simulink model "PV_MPPT"  (Simulink 10.0)
settings: Solver=ode23s  StartTime=0.0  StopTime=10  RelTol=1e-3  EnableMultiTasking=on
libraries: powerlib x12, powerlib_extras x2, simulink x1
settings Model: Creator=Administrator  LastModifiedBy=bhisma
settings SolverCC: ZeroCrossAlgorithm=Non-adaptive
settings DataIOCC: LimitDataPoints=on  SignalLoggingSaveFormat=ModelDataLogs
settings OptimizationCC: ExpressionDepthLimit=2147483647  InitFltsAndDblsToZero=on
settings DebuggingCC: SaveWithParameterizedLinksMsg=none  SolverPrmCheckMsg=warning  FcnCallInpInsideContextMsg=warning  StateNameClashWarn=warning
settings SFSimCC: SimUseLocalCustomCode=on  SimParseCustomCode=off  CustomCodeUndefinedFunction=FilterOut
settings RTWCC: RTWUseLocalCustomCode=on

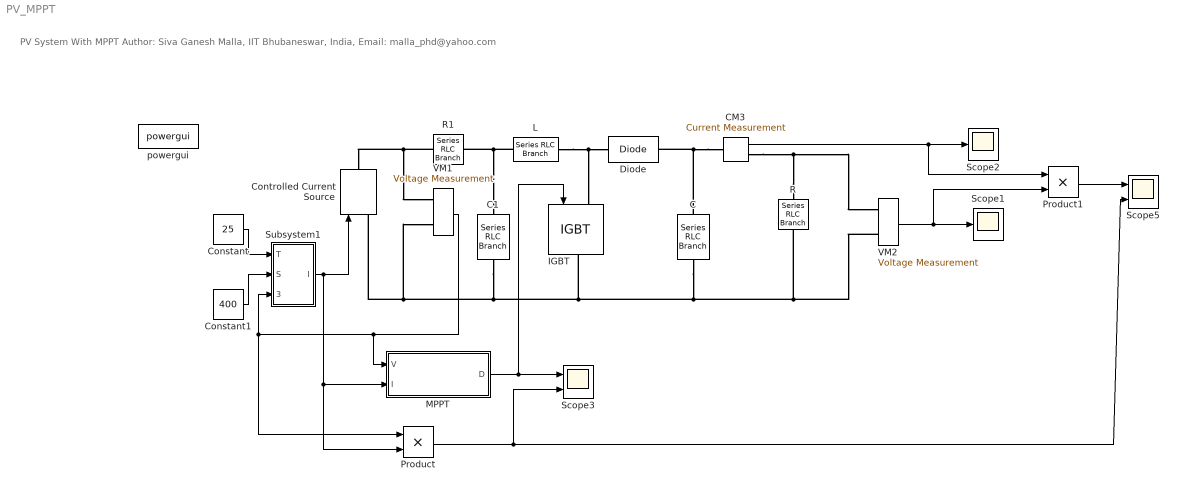
== system PV_MPPT ==
  note: PV System With MPPT
      | Author: Siva Ganesh Malla, IIT Bhubaneswar, India, Email: malla_phd@yahoo.com
  C : powerlib/Elements/Series RLC Branch  PhysicalDomain=powersysdomain  SubClassName=unknown  LeftPortType=p1  RightPortType=p1  LConnTagsString=__new0  RConnTagsString=__new0  BranchType=C  Resistance=0.01  Inductance=1.0  SetiL0=off  InitialCurrent=0  Capacitance=2e-3  Setx0=off  InitialVoltage=200  Measurements=None
      settings: SourceProductName=Simscape Electrical
  C1 : powerlib/Elements/Series RLC Branch  PhysicalDomain=powersysdomain  SubClassName=unknown  LeftPortType=p1  RightPortType=p1  LConnTagsString=__new0  RConnTagsString=__new0  BranchType=C  Resistance=0.01  Inductance=1.0  SetiL0=off  InitialCurrent=0  Capacitance=2e-3  Setx0=off  InitialVoltage=0  Measurements=None
      settings: SourceProductName=Simscape Electrical
  CM3 : powerlib/Measurements/Current Measurement  Tag=PoWeRsYsTeMmEaSuReMeNt  SystemSampleTime=-1  PhasorSimulation=off  OutputType=Magnitude  PSBequivalent=0
      settings: SourceProductName=Simscape Electrical
  Constant : Constant  Value=25
  Constant1 : Constant  Value=400
  Controlled Current Source : powerlib/Electrical Sources/Controlled Current Source  SystemSampleTime=-1  Initialize=on  Source_Type=AC  Amplitude=0  Phase=0  Frequency=0  Measurements=None
      settings: SourceProductName=Simscape Electrical
  Diode : powerlib/Power Electronics/Diode  SystemSampleTime=-1  Ron=0.001  Lon=0  Vf=0.8  IC=0  UseSnubber=off  Rs=500  Cs=250e-9  Measurements=off
      settings: SourceProductName=Simscape Electrical
  IGBT : powerlib/Power Electronics/IGBT  SystemSampleTime=-1  Ron=0.001  Lon=0  Vf=1  Tf=1e-6  Tt=2e-6  IC=0  Rs=1e5  Cs=inf  Measurements=off
      settings: SourceProductName=Simscape Electrical
  L : powerlib/Elements/Series RLC Branch  PhysicalDomain=powersysdomain  SubClassName=unknown  LeftPortType=p1  RightPortType=p1  LConnTagsString=__new0  RConnTagsString=__new0  BranchType=L  Resistance=1.0  Inductance=0.01  SetiL0=off  InitialCurrent=0  Capacitance=1.0  Setx0=off  InitialVoltage=0  Measurements=None
      settings: SourceProductName=Simscape Electrical
  MPPT : Subsystem
  Product : Product  RndMeth=Zero
  Product1 : Product  RndMeth=Zero
  R : powerlib/Elements/Series RLC Branch  PhysicalDomain=powersysdomain  SubClassName=unknown  LeftPortType=p1  RightPortType=p1  LConnTagsString=__new0  RConnTagsString=__new0  BranchType=R  Resistance=500  Inductance=1.0  SetiL0=off  InitialCurrent=0  Capacitance=1.0  Setx0=off  InitialVoltage=0  Measurements=None
      settings: SourceProductName=Simscape Electrical
  R1 : powerlib/Elements/Series RLC Branch  PhysicalDomain=powersysdomain  SubClassName=unknown  LeftPortType=p1  RightPortType=p1  LConnTagsString=__new0  RConnTagsString=__new0  BranchType=R  Resistance=1  Inductance=1.0  SetiL0=off  InitialCurrent=0  Capacitance=1.0  Setx0=off  InitialVoltage=0  Measurements=None
      settings: SourceProductName=Simscape Electrical
  Scope1 : Scope
  Scope2 : Scope
  Scope3 : Scope  NumInputPorts=2
  Scope5 : Scope  NumInputPorts=2
  Subsystem1 : Subsystem
  VM1 : powerlib/Measurements/Voltage Measurement  Tag=PoWeRsYsTeMmEaSuReMeNt  SystemSampleTime=-1  PhasorSimulation=off  OutputType=Magnitude  PSBequivalent=0
      settings: SourceProductName=Simscape Electrical
  VM2 : powerlib/Measurements/Voltage Measurement  Tag=PoWeRsYsTeMmEaSuReMeNt  SystemSampleTime=-1  PhasorSimulation=off  OutputType=Magnitude  PSBequivalent=0
      settings: SourceProductName=Simscape Electrical
  powergui : powerlib/powergui  SystemSampleTime=-1  SimulationMode=Continuous  SampleTime=50e-6  frequency=60  SPID=off  SwTol=0  Interpol=off  x0status=blocks  echomessages=off  HookPort=off  FunctionMessages=off  EnableUseOfTLC=off  RestoreLinks=warning  frequencyindice=0  Frange=[0:2:500]  Ylog=off  Xlog=on  ShowGrid=off  save=off  variable=ZData  ZoomFFT=on  StartTime=0.0  cycles=1  DisplayStyle=1  fundamental=60  FreqAxis=off  MaxFrequency=1000  frequencyindicesteady=1  RmsSteady=1  display=off  Ts=0  methode=off
      settings: SourceProductName=Simscape Electrical
  wires:
  Constant/1 -> Subsystem1/1(T)
  Subsystem1/1(I) -> Controlled Current Source/1, MPPT/2(I), Product/2
  CM3/1 -> Scope2/1, Product1/1
  VM2/1 -> Scope1/1, Product1/2
  VM1/1 -> Subsystem1/3(Uout), Product/1, MPPT/1(V)
  Product/1 -> Scope3/2, Scope5/2
  MPPT/1(D) -> IGBT/1, Scope3/1
  Constant1/1 -> Subsystem1/2(S)
  Product1/1 -> Scope5/1
  connections:
  C/RConn1 -- VM2/LConn2 -- R/RConn1 -- IGBT/RConn1 -- C1/RConn1 -- Controlled Current Source/LConn1 -- VM1/LConn2
  CM3/LConn1 -- C/LConn1 -- Diode/RConn1
  L/RConn1 -- Diode/LConn1 -- IGBT/LConn1
  R/LConn1 -- CM3/RConn1 -- VM2/LConn1
  R1/RConn1 -- Controlled Current Source/RConn1 -- VM1/LConn1
  L/LConn1 -- R1/LConn1 -- C1/LConn1

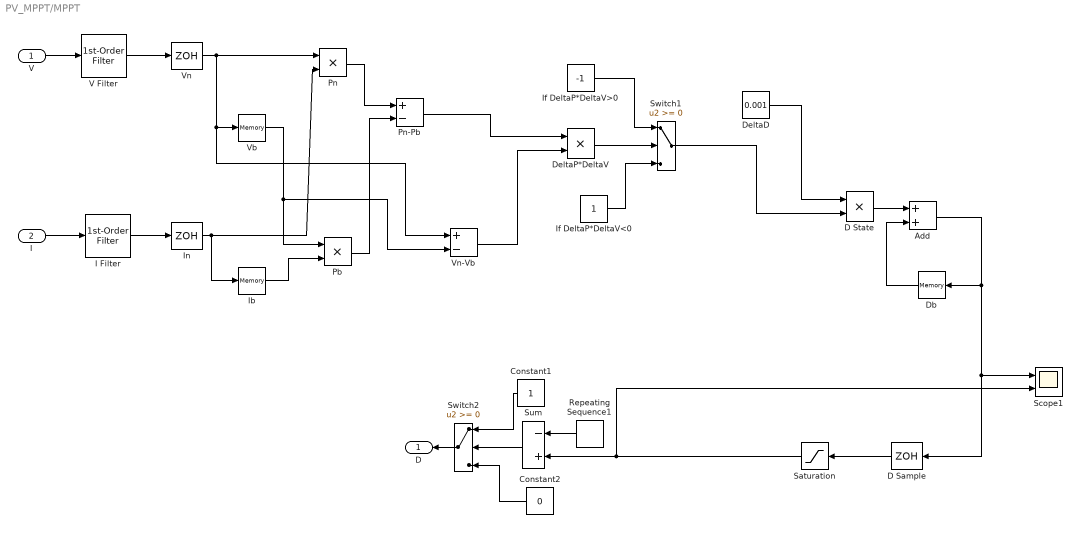
== system PV_MPPT/MPPT ==
  V : Inport
  I : Inport  Port=2
  Add : Sum
  Constant1 : Constant  SampleTime=-1
  Constant2 : Constant  Value=0  SampleTime=-1
  D Sample : ZeroOrderHold  SampleTime=1e-4
  D State : Product  RndMeth=Zero
  Db : Memory  InheritSampleTime=on  LinearizeAsDelay=on
  DeltaD : Constant  Value=0.001
  DeltaP*DeltaV : Product  RndMeth=Zero
  I Filter : powerlib_extras/Control  Blocks/1st-Order  Filter  SystemSampleTime=-1  FilterType=Lowpass  Tc=1e-3  Initialize=off  Vac_Init=[0.8 -25 60]  Vdc_Init=-0.4  PlotResponse=off  param1=[1 500 1]
      settings: SourceProductName=Simscape Electrical  SourceProductBaseCode=PS
  Ib : Memory  InheritSampleTime=on  LinearizeAsDelay=on
  If DeltaP*DeltaV<0 : Constant
  If DeltaP*DeltaV>0 : Constant  Value=-1
  In : ZeroOrderHold  SampleTime=1e-4
  Pb : Product  RndMeth=Zero
  Pn : Product  RndMeth=Zero
  Pn-Pb : Sum  Inputs=+-
  Repeating Sequence1 : simulink/Sources/Repeating Sequence  SystemSampleTime=-1  rep_seq_t=[0 4e-3 4e-3]  rep_seq_y=[0 1 0]
  Saturation : Saturate  UpperLimit=0.8  LowerLimit=0
  Scope1 : Scope  NumInputPorts=2
  Sum : Sum  Inputs=-+  SaturateOnIntegerOverflow=on
  Switch1 : Switch
  Switch2 : Switch
  V Filter : powerlib_extras/Control  Blocks/1st-Order  Filter  SystemSampleTime=-1  FilterType=Lowpass  Tc=1e-3  Initialize=off  Vac_Init=[0.8 -25 60]  Vdc_Init=-0.4  PlotResponse=off  param1=[1 500 1]
      settings: SourceProductName=Simscape Electrical  SourceProductBaseCode=PS
  Vb : Memory  InheritSampleTime=on  LinearizeAsDelay=on
  Vn : ZeroOrderHold  SampleTime=1e-4
  Vn-Vb : Sum  Inputs=+-
  D : Outport
  wires:
  V/1 -> V Filter/1
  I/1 -> I Filter/1
  V Filter/1 -> Vn/1
  I Filter/1 -> In/1
  In/1 -> Ib/1, Pn/2
  Vn/1 -> Pn/1, Vb/1, Vn-Vb/1
  Ib/1 -> Pb/2
  Vb/1 -> Pb/1, Vn-Vb/2
  Pn/1 -> Pn-Pb/1
  Pb/1 -> Pn-Pb/2
  D State/1 -> Add/1
  Constant2/1 -> Switch2/3
  Constant1/1 -> Switch2/1
  Sum/1 -> Switch2/2
  Repeating Sequence1/1 -> Sum/1
  Add/1 -> Db/1, D Sample/1, Scope1/1
  Switch2/1 -> D/1
  Db/1 -> Add/2
  D Sample/1 -> Saturation/1
  Pn-Pb/1 -> DeltaP*DeltaV/1
  Vn-Vb/1 -> DeltaP*DeltaV/2
  DeltaP*DeltaV/1 -> Switch1/2
  If DeltaP*DeltaV>0/1 -> Switch1/1
  If DeltaP*DeltaV<0/1 -> Switch1/3
  Switch1/1 -> D State/2
  DeltaD/1 -> D State/1
  Saturation/1 -> Sum/2, Scope1/2

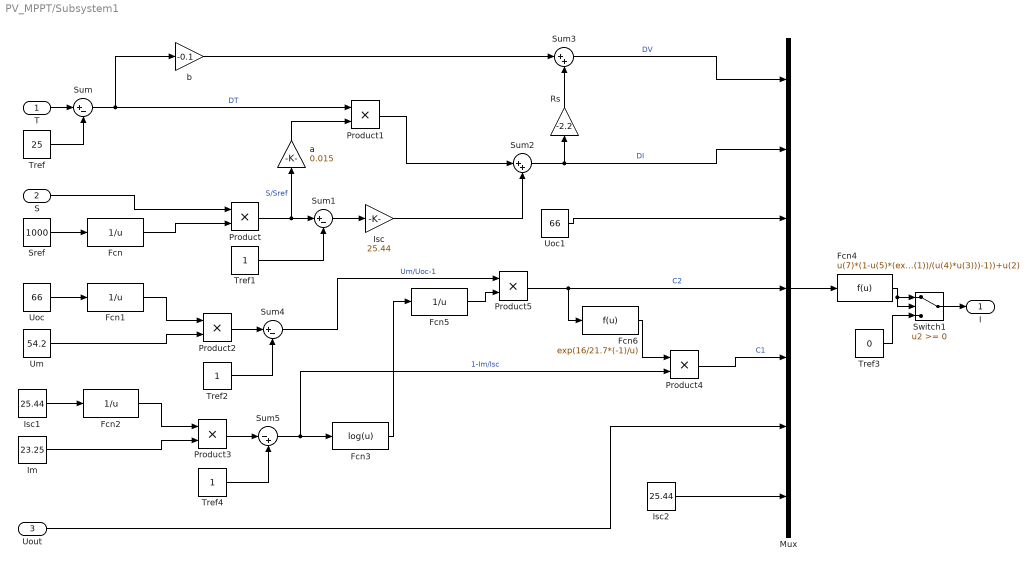
== system PV_MPPT/Subsystem1 ==
  T : Inport
  S : Inport  Port=2
  Uout : Inport  Port=3
  Fcn{,1..2,5} (4 alike) : Fcn  Expr=1/u
  Fcn3 : Fcn  Expr=log(u)
  Fcn4 : Fcn  Expr=u(7)*(1-u(5)*(exp((u(6)-u(1))/(u(4)*u(3)))-1))+u(2)
  Fcn6 : Fcn  Expr=exp(16/21.7*(-1)/u)
  Im : Constant  Value=23.25
  Isc : Gain  Gain=25.44
  Isc1 : Constant  Value=25.44
  Isc2 : Constant  Value=25.44
  Mux : Mux  Inputs=7
  Product{,1..5} (6 alike) : Product  RndMeth=Zero
  Rs : Gain  Gain=-2.2
  Sref : Constant  Value=1000
  Sum : Sum  Inputs=|+-
  Sum1 : Sum  Inputs=|+-
  Sum2 : Sum  Inputs=|++
  Sum3 : Sum  Inputs=|++
  Sum4 : Sum  Inputs=|+-
  Sum5 : Sum  Inputs=|-+
  Switch1 : Switch
  Tref : Constant  Value=25
  Tref1 : Constant
  Tref2 : Constant
  Tref3 : Constant  Value=0
  Tref4 : Constant
  Um : Constant  Value=54.2
  Uoc : Constant  Value=66
  Uoc1 : Constant  Value=66
  a : Gain  Gain=0.015
  b : Gain  Gain=-0.1
  I : Outport
  wires:
  T/1 -> Sum/1
  Tref/1 -> Sum/2
  Sum/1 -> Product1/1, b/1  "DT"
  Sref/1 -> Fcn/1
  Fcn/1 -> Product/2
  S/1 -> Product/1
  Product/1 -> Sum1/1, a/1  "S/Sref"
  Tref1/1 -> Sum1/2
  Sum1/1 -> Isc/1
  a/1 -> Product1/2
  Product1/1 -> Sum2/1
  Isc/1 -> Sum2/2
  Sum2/1 -> Rs/1, Mux/2  "DI"
  b/1 -> Sum3/1
  Rs/1 -> Sum3/2
  Sum3/1 -> Mux/1  "DV"
  Uoc/1 -> Fcn1/1
  Fcn1/1 -> Product2/1
  Um/1 -> Product2/2
  Product2/1 -> Sum4/1
  Tref2/1 -> Sum4/2
  Isc1/1 -> Fcn2/1
  Fcn2/1 -> Product3/1
  Im/1 -> Product3/2
  Product3/1 -> Sum5/1
  Tref4/1 -> Sum5/2
  Sum5/1 -> Fcn3/1, Product4/2  "1-Im/Isc"
  Mux/1 -> Fcn4/1
  Uoc1/1 -> Mux/3
  Uout/1 -> Mux/6
  Isc2/1 -> Mux/7
  Product5/1 -> Mux/4, Fcn6/1  "C2"
  Sum4/1 -> Product5/1  "Um/Uoc-1"
  Fcn3/1 -> Fcn5/1
  Fcn5/1 -> Product5/2
  Fcn6/1 -> Product4/1
  Product4/1 -> Mux/5  "C1"
  Tref3/1 -> Switch1/3
  Fcn4/1 -> Switch1/1, Switch1/2
  Switch1/1 -> I/1
